simulink model "Simulate_equation"  (R2020b)
settings: Solver=VariableStepAuto  StartTime=0.0  StopTime=10.0  RelTol=1e-3
PreLoadFcn:
  | t = [1 2 3 4 5];
model workspace (MAT data in the model file):
  C = 1e-05
  R = 10
  t = [1 2 3 4 5]
libraries: pid_lib x1
settings Model: Creator=user  LastModifiedBy=user

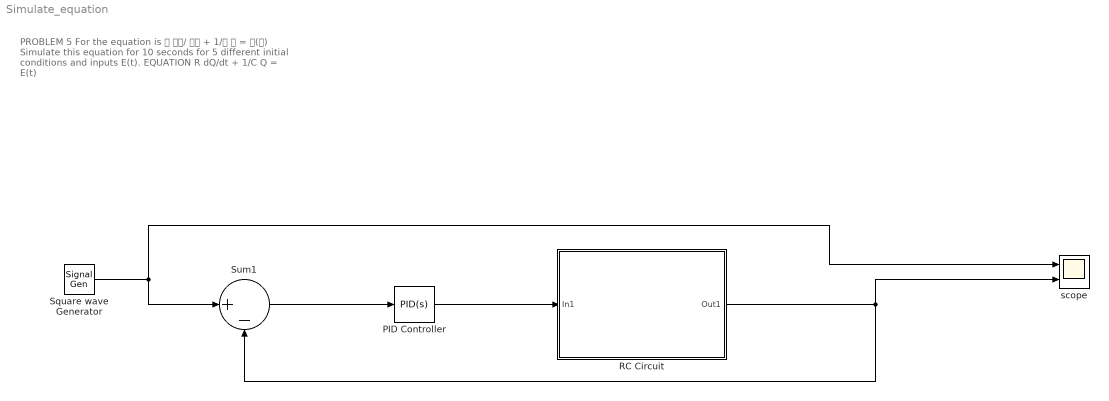
== system Simulate_equation ==
  note: PROBLEM 5
      |
      | For the equation is 𝑅 𝑑𝑄/ 𝑑𝑡 + 1/𝐶 𝑄 = 𝐸(𝑡) Simulate this equation for 10 seconds for 5 different initial conditions and inputs E(t).
      |
      | EQUATION
      | R dQ/dt + 1/C Q = E(t)
  PID Controller : pid_lib/PID Controller  Controller=PID  Form=Parallel  TimeDomain=Continuous-time  UseExternalTs=off  SampleTime=-1  IntegratorMethod=Forward Euler  FilterMethod=Forward Euler  ControllerParametersSource=internal  P=1  I=1  D=0  UseFilter=on  N=100  TunerSelectOption=Transfer Function Based (PID Tuner App)  InitialConditionSource=internal  InitialConditionForIntegrator=0  InitialConditionForFilter=0  DifferentiatorICPrevScaledInput=0  ExternalReset=none  TrackingMode=off  Kt=1  LimitOutput=off  SatLimitsSource=internal  UpperSaturationLimit=inf  LowerSaturationLimit=-inf  LinearizeAsGain=on  AntiWindupMode=none  Kb=1  POutMin=[]  POutMax=[]  IOutMin=[]  IOutMax=[]  DOutMin=[]  DOutMax=[]  NOutMin=[]  NOutMax=[]  SumOutMin=[]  SumOutMax=[]  SaturationOutMin=[]  SaturationOutMax=[]  PParamMin=[]  PParamMax=[]  IParamMin=[]  IParamMax=[]  DParamMin=[]  DParamMax=[]  NParamMin=[]  NParamMax=[]  KbParamMin=[]  KbParamMax=[]  KtParamMin=[]  KtParamMax=[]  KbOutMin=[]  KbOutMax=[]  KtOutMin=[]  KtOutMax=[]  IntegratorOutMin=[]  IntegratorOutMax=[]  FilterOutMin=[]  FilterOutMax=[]  SumI1OutMin=[]  SumI1OutMax=[]  SumI2OutMin=[]  SumI2OutMax=[]  SumI3OutMin=[]  SumI3OutMax=[]  SumI4OutMin=[]  SumI4OutMax=[]  SumDOutMin=[]  SumDOutMax=[]  DifferentiatorOutMin=[]  DifferentiatorOutMax=[]  FilterDiffOutCoefMin=[]  FilterDiffOutCoefMax=[]  ReciprocalOutMin=[]  ReciprocalOutMax=[]  SumDenOutMin=[]  SumDenOutMax=[]  SumNumOutMin=[]  SumNumOutMax=[]  DivideOutMin=[]  DivideOutMax=[]  UdiffTsProdOutMin=[]  UdiffTsProdOutMax=[]  NTsProdOutMin=[]  NTsProdOutMax=[]  UintegralTsProdOutMin=[]  UintegralTsProdOutMax=[]  UngainTsProdOutMin=[]  UngainTsProdOutMax=[]  IntegratorContinuousStateAttributes=''  IntegratorStateMustResolveToSignalObject=off  IntegratorRTWStateStorageClass=Auto  FilterContinuousStateAttributes=''  FilterStateMustResolveToSignalObject=off  FilterRTWStateStorageClass=Auto  ParallelPVariant=InternalParameters  IdealPVariant=Disabled  IVariant=InternalParameters  DVariant=InternalParameters  IntegratorVariant=Continuous  SatVariant=Disabled  AWVariant=Passthrough  PCopyVariant=Disabled  TRVariant=Disabled  FdbkBlocksVariant=Forward  IdealPFdbkVariant=Disabled  SatFdbkVariant=Disabled  DerivativeFilterVariant=ContFilter  NVariant=InternalParameters  NCopyVariant=Disabled  FilterICVariant=InternalICsFilter  IntegratorICVariant=InternalICs  ExternalResetVariant=Disabled  TRSumVariant=Passthrough  SumFdbkVariant=Disabled  SumVariant=Sum_PID  TsampFilterVariant=InternalTs  TsampNgainVariant=Passthrough  TsampIntegralVariant=Passthrough  ExternalSaturationOutDataTypeStr=Inherit: Same as second input
  RC Circuit : Subsystem  mask{R=10, C=10*10^-6, q_init=0}
      mask prompts: R "Resistance"; C "Capacitance"; q_init "Initial charge capacitor"
      mask Display: image('C:\Users\user\Desktop\MBD Milestone\Problem 5\Mask icon Image\RC_circuit.jpg'); % Use "Edit Image" on toolstrip to change.
  Square wave Generator : SignalGenerator  WaveForm=square  Amplitude=t  Units=rad/sec
  Sum1 : Sum  Inputs=|+-
  scope : Scope  NumInputPorts=2
  wires:
  Sum1/1 -> PID Controller/1
  PID Controller/1 -> RC Circuit/1(In1)
  Square wave Generator/1 -> scope/1, Sum1/1
  RC Circuit/1(Out1) -> scope/2, Sum1/2

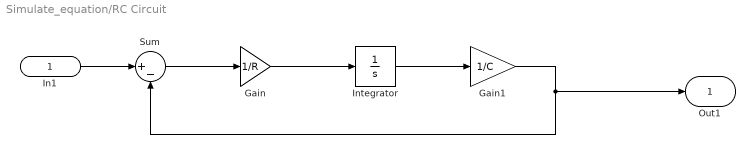
== system Simulate_equation/RC Circuit ==
  In1 : Inport
  Gain : Gain  Gain=1/R
  Gain1 : Gain  Gain=1/C
  Integrator : Integrator  InitialCondition=q_init
  Sum : Sum  Inputs=|+-
  Out1 : Outport
  wires:
  Gain/1 -> Integrator/1
  In1/1 -> Sum/1
  Integrator/1 -> Gain1/1
  Gain1/1 -> Sum/2, Out1/1
  Sum/1 -> Gain/1
